simulink model "AMDSBProject"  (R2020b)
settings: Solver=VariableStepAuto  StartTime=0.0  StopTime=10.0  RelTol=1e-3
libraries: commchan3 x1, dsparch4 x1
settings Model: Creator=gideon  LastModifiedBy=gideon

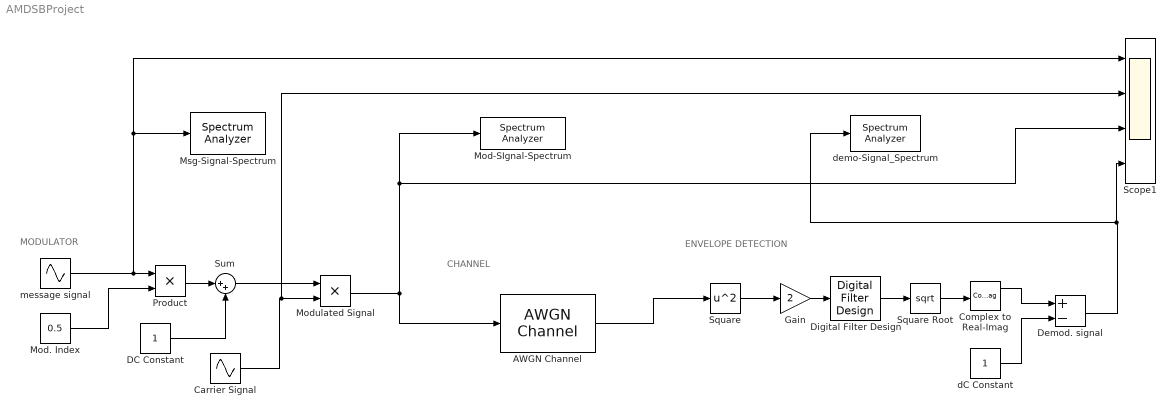
== system AMDSBProject ==
  note: ENVELOPE DETECTION
  note: MODULATOR
  note: CHANNEL
  AWGN Channel : commchan3/AWGN Channel  InputProcessing=Columns as channels (frame based)  seed=1  noiseMode="Signal to noise ratio  (SNR)"  EbNodB=20  EsNodB=10  SNRdB=10  bitsPerSym=64  Ps=1  Tsym=1e-4  variance=1
  Carrier Signal : Sin  Amplitude=1.5  Frequency=2*pi*8000  Phase=pi / 2  SampleTime=1/48000
  Complex to Real-Imag : ComplexToRealImag
  DC Constant : Constant
  Demod. signal : Sum  Inputs=+-
  Digital Filter Design : dsparch4/Digital Filter Design  mwdsp_browser_bugfix_var=off
  Gain : Gain  Gain=2
  "Mod-SIgnal-Spectrum " : SpectrumAnalyzer
  Mod. Index : Constant  Value=0.5
  Modulated Signal : Product
  Msg-Signal-Spectrum : SpectrumAnalyzer
  Product : Product
  Scope1 : Scope  NumInputPorts=4
  Square : Math  Operator=square  SaturateOnIntegerOverflow=on
  Square Root : Sqrt  OutputSignalType=complex  RndMeth=Round  SaturateOnIntegerOverflow=on
  Sum : Sum  Inputs=|++
  dC Constant : Constant
  demo-Signal_Spectrum : SpectrumAnalyzer
  message signal : Sin  Frequency=2*pi*1000  SampleTime=1/48000
  wires:
  DC Constant/1 -> Sum/2
  Complex to Real-Imag/1 -> Demod. signal/1
  Mod. Index/1 -> Product/2
  Product/1 -> Sum/1
  Carrier Signal/1 -> Modulated Signal/2, Scope1/2
  dC Constant/1 -> Demod. signal/2
  Digital Filter Design/1 -> Square Root/1
  Square Root/1 -> Complex to Real-Imag/1
  AWGN Channel/1 -> Square/1
  message signal/1 -> Scope1/1, Msg-Signal-Spectrum/1, Product/1
  Square/1 -> Gain/1
  Modulated Signal/1 -> Scope1/3, "Mod-SIgnal-Spectrum "/1, AWGN Channel/1
  Gain/1 -> Digital Filter Design/1
  Sum/1 -> Modulated Signal/1
  Demod. signal/1 -> demo-Signal_Spectrum/1, Scope1/4
